simulink library "dspsnks4"  (Simulink 8.1)
settings: Solver=ode45  SolverMode=SingleTasking  StartTime=0.0  StopTime=10.0  RelTol=1e-3
undefined symbols (not defined in the file or in its folder): sdspwfall
undefined symbols (not defined in the file): get, hot
libraries: dspvision x1, dspnetwork x1
settings Model: RequirementInfo=9  FPTRunName=Active  ForwardingTableString=||__slOldName__||dspsnks4/To Wave File||__slNewName__||dspwin32/To Wave File||__slOldName__||dspsnks4/Spectrum Scope||__slNewName__||dspsnks4/Spectrum Analyzer||__slOldName__||dspsnks4/To Multimedia File||__slNewName__||dspvision/To Multimedia File  Creator=don  LastModifiedBy=dsomasun  CovMetricSettings=d  ExtModeAutoUpdateStatusClock=off

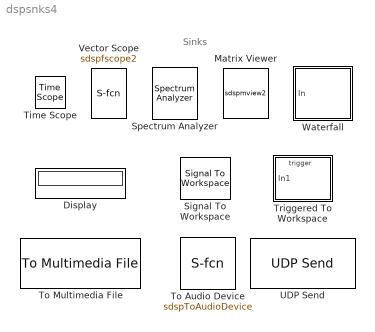
== system dspsnks4 ==
  note: Sinks
  Display : Display
  Matrix Viewer : M-S-Function  DialogController=dspdialog.MatrixViewer  DialogControllerArgs=DataTag0  FunctionName=sdspmview2  Parameters={CMapStr},YMin,YMax,AxisColorbar,AxisOrigin,{XLabel},{YLabel},{ZLabel},FigPos,AxisZoom  DisplayMFileStacktrace=off  mask(Matrix Viewer){ShowPortLabels=off, ImageParams=off, CMapStr=hot(256), YMin=-1.0, YMax=1.0, AxisColorbar=on, AxisParams=off, AxisOrigin=Upper left corner, XLabel=X-axis, YLabel=Y-axis, ZLabel=Z-axis, FigPos=get(0,'defaultfigureposition'), AxisZoom=off}
      mask prompts: ShowPortLabels "dummy"; ImageParams "-------------------------------- Show Image properties ------------------------------------"; CMapStr "Colormap matrix:"; YMin "Minimum input value:"; YMax "Maximum input value:"; AxisColorbar "Display colorbar"; AxisParams "-------------------------------- Show axis properties ----------------------------------------"; AxisOrigin "Axis origin:"; XLabel "X-axis title:"; YLabel "Y-axis title:"; ZLabel "Colorbar title:"; FigPos "Figure position:"; AxisZoom "Axis zoom"
      mask help: Display a matrix as an image, scaling the colormap to the specified input data range. Colormap must be an Nx3 matrix of RGB values. Type "help graph3d" at the MATLAB prompt for a list of predefined colormaps.
      settings: CopyFcn=sdspmview2([],[],[],'BlockCopy');  DeleteFcn=sdspmview2([],[],[],'BlockDelete');  NameChangeFcn=sdspmview2([],[],[],'BlockNameChange');
      mask Help: eval('blocksethelp');
      mask TypeOptions AxisOrigin: Upper left corner | Lower left corner
      mask Display: disp('Matrix\nViewer')
  Signal To Workspace : SignalToWorkspace  VariableName=yout
      settings: CopyFcn=dspblkcopystw(gcbh);
  Spectrum Analyzer : SpectrumAnalyzer
  Time Scope : TimeScope  DefaultConfigurationName=spbscopes.TimeScopeBlockCfg
  To Audio Device : S-Function  DialogController=dspDDGCreate  DialogControllerArgs=DataTag1  FunctionName=sdspToAudioDevice  Parameters=deviceName, inheritSampleRate, sampleRate, deviceDatatype, autoBufferSize, bufferSize, queueDuration,defaultOutputChannelMapping,outputChannelMapping  EnableBusSupport=off  mask(To Audio Device){deviceName=Default, inheritSampleRate=on, sampleRate=44100, deviceDatatype=Determine from input data type, autoBufferSize=on, bufferSize=4096, queueDuration=1.0, defaultOutputChannelMapping=on, outputChannelMapping=1}
      mask prompts: deviceName "Device name"; inheritSampleRate "Inherit sample rate"; sampleRate "Sample rate (Hz)"; deviceDatatype "Device data type"; autoBufferSize "Automatically determine buffer size"; bufferSize "Buffer size (samples)"; queueDuration "Queue duration (seconds)"; defaultOutputChannelMapping "Use default mapping between Data and Device Output Channels"; outputChannelMapping "Device Output Channels"
      mask help: Send sound data to your computer's audio device.
      mask init:
      | icon = dspdialog.ToAudioDevice.maskInit();
      mask Help: eval('blocksethelp');
      mask TypeOptions deviceDatatype: Determine from input data type | 8-bit integer | 16-bit integer | 24-bit integer | 32-bit float
      mask Display:
      | patch(icon.x1, icon.y1,[1 1 1]*.5);
      | patch(icon.x2, icon.y2);
      | plot(icon.x, icon.y);
      | plot(icon.x1, icon.y1);
  To Multimedia File : dspvision/To Multimedia File  outputFilename=output.wav  streamSelection=Audio only  videoCompressor=None (uncompressed)  audioCompressor=None (uncompressed)  imagePorts=Separate color signals  fileType=WAV  audioDatatype=16-bit integer  fourcc=RGB
  Triggered To Workspace : Subsystem  TreatAsAtomicUnit=on  mask(Triggered To Workspace){TriggerType=Rising edge, VariableName=yout, Buffer=1000, Decimation=1, Save2DMode=2-D array (concatenate along first dimension), FixptAsFi=off}
      mask prompts: TriggerType "Trigger type:"; VariableName "Variable name:"; Buffer "Maximum number of rows:"; Save2DMode "Save 2-D signals as:"; FixptAsFi "Log fixed-point data as a fi object"
      mask help: Write input to specified variable in the workspace when trigger is received.
      mask init:
      | dspblktrigtwks('init',TriggerType);
      settings: CopyFcn=dspblkcopystw(gcbh);
      mask Help: eval('blocksethelp');
      mask TypeOptions TriggerType: Rising edge | Falling edge | Either edge
      mask TypeOptions Save2DMode: 2-D array (concatenate along first dimension) | 3-D array (concatenate along third dimension) | Inherit from input (this choice will be removed - see release notes)
      mask Display: disp(VariableName);
  UDP Send : dspnetwork/UDP Send  remoteURL='127.0.0.1'  remotePort=25000  localURL='0.0.0.0'  localPortSource=Automatically determine  localPort=-1  sampletime=-1  separateLengthPort=0
  Vector Scope : M-S-Function  DialogController=dspdialog.VectorScope  DialogControllerArgs=DataTag3  FunctionName=sdspfscope2  Parameters=1  DisplayMFileStacktrace=off  mask(Vector Scope){ScopeProperties=on, Domain=Time, HorizSpan=1, DisplayProperties=off, AxisGrid=on, Memory=off, FrameNumber=on, AxisLegend=off, AxisZoom=off, OpenScopeAtSimStart=on, OpenScopeImmediately=off, FigPos=get(0,'defaultfigureposition'), AxisProperties=off, XUnits=Hertz, XRange=[0...Fs/2], InheritXIncr=on, XIncr=1, XLabel=Time, XLimit=Auto, XMin=0, XMax=1, XStart=0, YUnits=dB, YMin=-10, YMax=10, YLabel=Amplitude, LineProperties=off, LineDisables=, LineStyles=, LineMarkers=, LineColors=, ShowPortLabels=off, XAxisParamsVer=6.8}
      mask prompts: ScopeProperties "-------------------------------- Show scope properties ------------------------------------"; Domain "Input domain:"; HorizSpan "Time display span (number of frames):"; DisplayProperties "-------------------------------- Show display properties -----------------------------------"; AxisGrid "Show grid"; Memory "Persistence"; FrameNumber "Frame number"; AxisLegend "Channel legend"; AxisZoom "Compact display"; OpenScopeAtSimStart "Open scope at start of simulation"; OpenScopeImmediately "Open scope immediately"; FigPos "Scope position:"; AxisProperties "-------------------------------- Show axis properties ----------------------------------------"; XUnits "Frequency units:"; XRange "Frequency range:"; InheritXIncr "Inherit sample increment from input"; XIncr "Increment per sample in input frame:"; XLabel "X-axis title:"; XLimit "X limits:"; XMin "Minimum X-limit:"; XMax "Maximum X-limit:"; XStart "X Start"; YUnits "Amplitude scaling:"; YMin "Minimum Y-limit:"; YMax "Maximum Y-limit:"; YLabel "Y-axis title:"; LineProperties "-------------------------------- Show line properties -----------------------------------------"; LineDisables "Line visibilities:"; LineStyles "Line styles:"; LineMarkers "Line markers:"; LineColors "Line colors:"; ShowPortLabels "dummy"; XAxisParamsVer "Version of X-axis parameters:"
      mask help:
      | Display a vector or matrix of time-domain, frequency-domain, or user-specified data.  Each column of a 2-D input matrix is plotted as a separate data channel.  1-D inputs are assumed to be a single data channel.
      |
      | For frequency-domain operation, input should come from a source such as the Magnitude FFT block, or a block with equivalent data organization.
      mask init:
      | [x,y,str] = dspblkfscope2('icon');
      | s = dspblkfscope2('init');
      settings: DeleteFcn=sdspfscope2([],[],[],'BlockDelete');  NameChangeFcn=sdspfscope2([],[],[],'NameChange');
      settings: CopyFcn=|
      | sdspfscope2([],[],[],'BlockCopy');
      | set_param(gcb,'XAxisParamsVer','6.9');
      mask Help: eval('blocksethelp');
      mask TypeOptions Domain: Time | Frequency | User-defined
      mask TypeOptions XUnits: Hertz | rad/sec
      mask TypeOptions XRange: [0...Fs/2] | [-Fs/2...Fs/2] | [0...Fs]
      mask TypeOptions XLimit: Auto | User-defined
      mask TypeOptions YUnits: Magnitude | dB
      mask TypeOptions XAxisParamsVer: 6.8 | 6.9
      mask Display: plot(x,y); text(14,20,str);
  Waterfall : Subsystem  LoadFcn=sdspwfall([],[],[],'BlockLoad');  TreatAsAtomicUnit=on  SimViewingDevice=on  mask(Waterfall){TraceProperties=off, NumTraces=6, CMapStr=autumn, TNewest=1, TOldest=0, HistoryLength=10, HistoryFull=Overwrite, UpdateInterval=1, ExportMode=Selected, MLExportName=ExportData, AutoExport=off, DisplayProperties=off, MouseMode=Orbit, AxisGrid=on, Snapshot=off, Suspend=off, SyncSnapshots=off, OpenScopeAtSimStart=on, FigPos=[243 195 405 320], CameraView=[69.4600750684385 564.426060114276 -133.474523953492 0 18.5 3.5 0.616338299486424 -7.9078811427274 1.98411164834144 2.40985953613679 1 18.5 3], InportDimsHint=[32 1], AxisProperties=off, YMin=-1, YMax=1, AxisColor='w', XLabel=Amplitude, YLabel=Samples, ZLabel=Time, TriggerProperties=off, TrigStartMode=Immediately, TrigStartT=0, TrigStartN=0, TrigStartFcn=trigbegin, TrigStopMode=Never, TrigStopT=0.1, TrigStopN=1, TrigStopFcn=trigend, TrigRearmMode=Never, TrigRearmT=0, TrigRearmN=0, TrigRearmFcn=trigrearm, XformProperties=on, XformMode=None, XformFcn=abs, XformExpr=(u+1)/2}
      mask prompts: TraceProperties "-------------------------------- Show waterfall properties ------------------------------------"; NumTraces "Number of traces:"; CMapStr "Colormap name (jet, hot, etc):"; TNewest "Transparency of newest trace, 0 to 1 (1=opaque):"; TOldest "Transparency of oldest trace, 0 to 1:"; HistoryLength "History length:"; HistoryFull "History full:"; UpdateInterval "Display update interval:"; ExportMode "Data logging:"; MLExportName "MATLAB export variable name:"; AutoExport "Automatic export to workspace"; DisplayProperties "-------------------------------- Show display properties ----------------------------------------"; MouseMode "Mouse mode:"; AxisGrid "Show grid"; Snapshot "Snapshot (pause) display"; Suspend "Suspend data capture"; SyncSnapshots "Synchronize suspend/snapshot"; OpenScopeAtSimStart "Open scope at start of simulation"; FigPos "Scope position:"; CameraView "Camera view:"; InportDimsHint "Inport dimensions hint:"; AxisProperties "-------------------------------- Show axis properties ----------------------------------------"; YMin "Minimum input value:"; YMax "Maximum input value:"; AxisColor "Axis color:"; XLabel "X-axis title:"; YLabel "Y-axis title:"; ZLabel "Z-axis title:"; TriggerProperties "-------------------------------- Show trigger properties ----------------------------------------"; TrigStartMode "Begin recording:"; TrigStartT "Begin record time, T:"; TrigStartN "Begin record count, N:"; TrigStartFcn "Begin record function:"; TrigStopMode "Record until:"; TrigStopT "End record time, T:"; TrigStopN "End record count, N:"; TrigStopFcn "End record function:"; TrigRearmMode "Re-enable recording:"; TrigRearmT "Re-enable time, T:"; TrigRearmN "Re-enable count, N:"; TrigRearmFcn "Re-enable function:"; XformProperties "-------------------------------- Show transform properties ----------------------------------------"; XformMode "Transform:"; XformFcn "Function:"; XformExpr "Expression:"
      mask help:
      | Display sequence of vectors as a 3-D waterfall plot.  Input must be real-valued.  For matrix inputs, each column of data is treated as a sequential vector input to the waterfall.
      |
      | Colormap must be the name of a MATLAB colormap function, without arguments or parentheses.  Type "help graph3d" at the MATLAB prompt for a list of predefined colormaps.
      mask init:
      | if strcmp(Suspend,'on'),
      | 	str='Suspend';
      | elseif strcmp(Snapshot,'on'),
      | 	str='SnapShot';
      | else
      | 	str='';
      | end
      | sdspwfall([],[],[],'DialogApply');
      settings: CopyFcn=sdspwfall([],[],[],'BlockCopy');  DeleteFcn=sdspwfall([],[],[],'BlockDelete');  UndoDeleteFcn=sdspwfall([],[],[],'BlockUndoDelete');  NameChangeFcn=sdspwfall([],[],[],'BlockNameChange');  OpenFcn=sdspwfall([],[],[],'BlockOpen');  ErrorFcn=sdspwfall  RTWSystemCode=Non-reusable function
      mask Help: eval('blocksethelp');
      mask Callback TraceProperties: dspblkwfall('dynamic','TraceProperties');
      mask TypeOptions HistoryFull: Overwrite | Suspend | Extend
      mask TypeOptions ExportMode: Selected | All visible | All history
      mask Callback DisplayProperties: dspblkwfall('dynamic','DisplayProperties');
      mask TypeOptions MouseMode: Arrow | Orbit | Zoom
      mask Callback AxisProperties: dspblkwfall('dynamic','AxisProperties');
      mask Callback TriggerProperties: dspblkwfall('dynamic','TriggerProperties');
      mask TypeOptions TrigStartMode: Immediately | After T seconds | After N inputs | User-defined
      mask TypeOptions TrigStopMode: Never | After T seconds | After N inputs | User-defined
      mask TypeOptions TrigRearmMode: Never | After T seconds | After N inputs | User-defined
      mask Callback XformProperties: dspblkwfall('dynamic','XformProperties');
      mask TypeOptions XformMode: None | Amplitude->dB | Complex->Mag Lin | Complex->Mag dB | Complex->Angle | FFT->Mag Lin Fs/2 | FFT->Mag dB Fs/2 | FFT->Angle Fs/2 | Power->dB | User-defined fcn | User-defined expr
      mask Display:
      | disp('Waterfall\nScope\n')
      | color('red')
      | text(.08,.2,str)

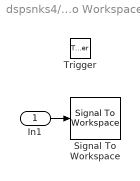
== system dspsnks4/Triggered To Workspace ==
  In1 : Inport
  Trigger : TriggerPort
  Signal To Workspace : SignalToWorkspace  VariableName=yout
      settings: CopyFcn=dspblkcopystw(gcbh);
  wires:
  In1/1 -> Signal To Workspace/1

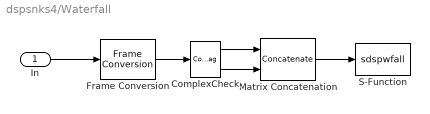
== system dspsnks4/Waterfall ==
  In : Inport
  ComplexCheck : ComplexToRealImag
  Frame Conversion : FrameConversion  OutFrame=Sample-based
  Matrix Concatenation : Concatenate  Mode=Multidimensional array
  S-Function : M-S-Function  FunctionName=sdspwfall  DisplayMFileStacktrace=off
  wires:
  Matrix Concatenation/1 -> S-Function/1
  ComplexCheck/2 -> Matrix Concatenation/2
  ComplexCheck/1 -> Matrix Concatenation/1
  In/1 -> Frame Conversion/1
  Frame Conversion/1 -> ComplexCheck/1
